simulink model "CONTROLLER_MOD"  (Simulink 5.0)
settings: Solver=ode45  StartTime=0.0  StopTime=10.0  RelTol=1e-3
settings Model: LastModifiedBy=Administrator

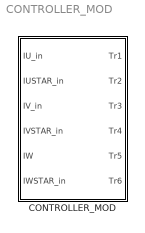
== system CONTROLLER_MOD ==
  CONTROLLER_MOD : Subsystem

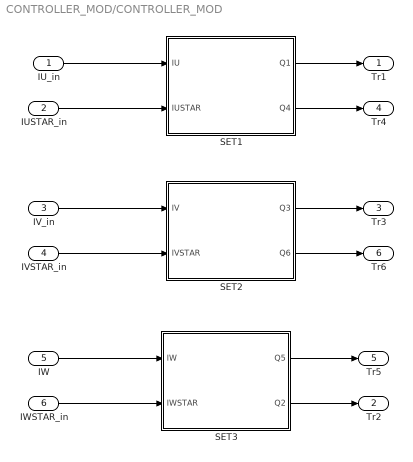
== system CONTROLLER_MOD/CONTROLLER_MOD ==
  IU_in : Inport
  IUSTAR_in : Inport  Port=2
  IV_in : Inport  Port=3
  IVSTAR_in : Inport  Port=4
  IW : Inport  Port=5
  IWSTAR_in : Inport  Port=6
  SET1 : Stateflow chart
  SET2 : Stateflow chart
  SET3 : Stateflow chart
  Tr1 : Outport
  Tr2 : Outport  Port=2
  Tr3 : Outport  Port=3
  Tr4 : Outport  Port=4
  Tr5 : Outport  Port=5
  Tr6 : Outport  Port=6
  wires:
  IU_in/1 -> SET1/1(IU)
  IUSTAR_in/1 -> SET1/2(IUSTAR)
  IV_in/1 -> SET2/1(IV)
  IVSTAR_in/1 -> SET2/2(IVSTAR)
  IW/1 -> SET3/1(IW)
  IWSTAR_in/1 -> SET3/2(IWSTAR)
  SET1/1(Q1) -> Tr1/1
  SET3/2(Q2) -> Tr2/1
  SET2/1(Q3) -> Tr3/1
  SET1/2(Q4) -> Tr4/1
  SET3/1(Q5) -> Tr5/1
  SET2/2(Q6) -> Tr6/1

== stateflow chart CONTROLLER_MOD/SET1 ==
  settings: updateMethod=CONTINUOUS  executeAtInitialization=1
  state A/
    state A1/
      during:Q1=1;Q4=0;
    state A2/
      during:Q4=1;Q1=0;
    A1 -> A2 : [IU>IUSTAR]
    A2 -> A1 : [IU<IUSTAR]
  (default) -> A : [1]
  data: IU input double; IUSTAR input double; Q1 output double; Q4 output double

== stateflow chart CONTROLLER_MOD/SET2 ==
  settings: updateMethod=CONTINUOUS  executeAtInitialization=1
  state B/
    state B1/
      during:Q1=1;Q4=0;
    state B2/
      during:Q4=1;Q1=0;
    B1 -> B2 : [IV>IVSTAR]
    B2 -> B1 : [IV<IVSTAR]
  (default) -> B : [1]
  data: IV input double; IVSTAR input double; Q3 output double; Q6 output double

== stateflow chart CONTROLLER_MOD/SET3 ==
  settings: updateMethod=CONTINUOUS  executeAtInitialization=1
  state C/
    state C1/
      during:Q1=1;Q4=0;
    state C2/
      during:Q4=1;Q1=0;
    C1 -> C2 : [IW>IWSTAR]
    C2 -> C1 : [IW<IWSTAR]
  (default) -> C : [1]
  data: IW input double; IWSTAR input double; Q5 output double; Q2 output double
